simulink model "Impedance"  (R2021a)
settings: Solver=VariableStepAuto  StartTime=0.0  StopTime=2  RelTol=1e-3
values from neighbouring files (symbols this model uses):
  kd = 2*z*w    [params.m]
  kp = w^2    [params.m]
  Md = eye(6)*100    [params.m]
  x = [ 0.5357 ... (first row only)    [params.m]
settings Model: Creator=Sebastiano  LastModifiedBy=antoninoparisi
settings SolverCC: AlgebraicLoopSolver=TrustRegion
settings DebuggingCC: SFMachineParentedDataDiag=warning

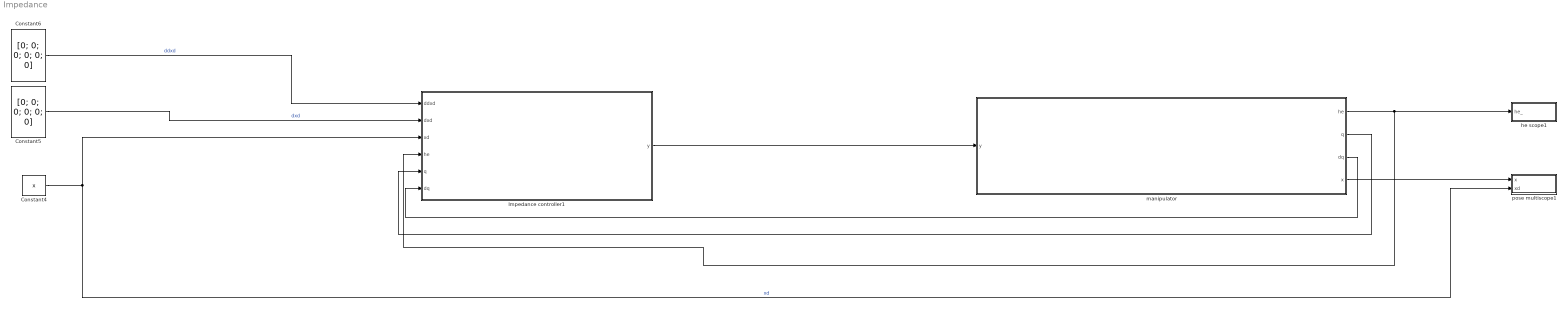
== system Impedance ==
  Constant4 : Constant  Value=x  VectorParams1D=off
  Constant5 : Constant  Value=[0; 0; 0; 0; 0; 0]  VectorParams1D=off
  Constant6 : Constant  Value=[0; 0; 0; 0; 0; 0]  VectorParams1D=off
  Impedance controller1 : Subsystem
  he scope1 : Subsystem
  manipulator : Subsystem
  pose multiscope1 : Subsystem
  wires:
  Constant5/1 -> Impedance controller1/2(dxd)  "dxd"
  manipulator/1(he) -> he scope1/1(he_), Impedance controller1/4(he)
  manipulator/3(dq) -> Impedance controller1/6(dq)
  Constant6/1 -> Impedance controller1/1(ddxd)  "ddxd"
  manipulator/2(q) -> Impedance controller1/5(q)
  manipulator/4(x) -> pose multiscope1/1(x)
  Constant4/1 -> Impedance controller1/3(xd), pose multiscope1/2(xd)  "xd"
  Impedance controller1/1(y) -> manipulator/1(y)

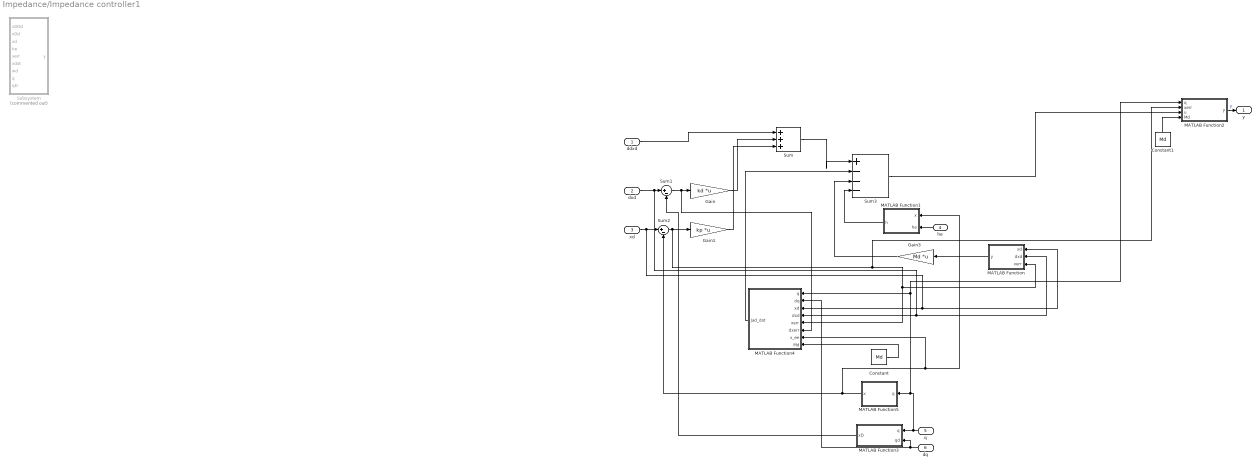
== system Impedance/Impedance controller1 ==
  ddxd : Inport
  dxd : Inport  Port=2
  xd : Inport  Port=3
  he : Inport  Port=4
  q : Inport  Port=5
  dq : Inport  Port=6
  Constant : Constant  Value=Md
  Constant1 : Constant  Value=Md
  Gain : Gain  Gain=kd  Multiplication=Matrix(K*u) (u vector)
  Gain1 : Gain  Gain=kp  Multiplication=Matrix(K*u) (u vector)
  Gain3 : Gain  Gain=Md  Multiplication=Matrix(K*u) (u vector)
  MATLAB Function : MATLAB Function  TreatAsAtomicUnit=on
  MATLAB Function1 : MATLAB Function  TreatAsAtomicUnit=on
  MATLAB Function2 : MATLAB Function  TreatAsAtomicUnit=on
  MATLAB Function3 : MATLAB Function  TreatAsAtomicUnit=on
  MATLAB Function4 : MATLAB Function  TreatAsAtomicUnit=on
  MATLAB Function5 : MATLAB Function  TreatAsAtomicUnit=on
  Subsystem : Subsystem  Commented=on
  Sum : Sum  Inputs=|+++
  Sum1 : Sum  Inputs=|+-
  Sum2 : Sum  Inputs=|+-
  Sum3 : Sum  Inputs=|+---
  y : Outport
  wires:
  xd/1 -> MATLAB Function/1(xd), MATLAB Function4/3(xd), Sum2/1
  Sum2/1 -> MATLAB Function/3(xerr), MATLAB Function4/5(xerr), MATLAB Function2/2(xerr), Gain1/1
  dxd/1 -> MATLAB Function/2(dxd), MATLAB Function4/4(dxd), Sum1/1
  Sum1/1 -> MATLAB Function4/6(dxerr), Gain/1
  ddxd/1 -> Sum/1
  Gain/1 -> Sum/2
  Gain1/1 -> Sum/3
  dq/1 -> MATLAB Function4/2(dq), MATLAB Function3/2(qd)
  q/1 -> MATLAB Function2/1(q), MATLAB Function4/1(q), MATLAB Function5/1(q), MATLAB Function3/1(q)
  MATLAB Function3/1(xD) -> Sum1/2
  MATLAB Function5/1(x) -> MATLAB Function4/7(x_ee), MATLAB Function1/1(x), Sum2/2
  Sum/1 -> Sum3/1
  Sum3/1 -> MATLAB Function2/3(u)
  MATLAB Function/1(y) -> Gain3/1
  MATLAB Function2/1(y) -> y/1  "y"
  MATLAB Function1/1(h) -> Sum3/4
  MATLAB Function4/1(Jad_dot) -> Sum3/2
  Gain3/1 -> Sum3/3
  he/1 -> MATLAB Function1/2(he)
  Constant/1 -> MATLAB Function4/8(Md)
  Constant1/1 -> MATLAB Function2/4(Md)

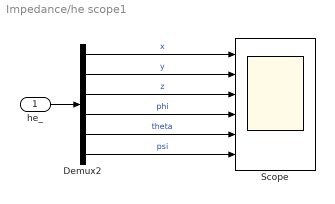
== system Impedance/he scope1 ==
  he_ : Inport
  Demux2 : Demux  Outputs=[1, 1, 1, 1, 1, 1]
  Scope : Scope  NumInputPorts=6
  wires:
  Demux2/4 -> Scope/4  "phi"
  Demux2/3 -> Scope/3  "z"
  Demux2/6 -> Scope/6  "psi"
  Demux2/5 -> Scope/5  "theta"
  Demux2/1 -> Scope/1  "x"
  he_/1 -> Demux2/1
  Demux2/2 -> Scope/2  "y"

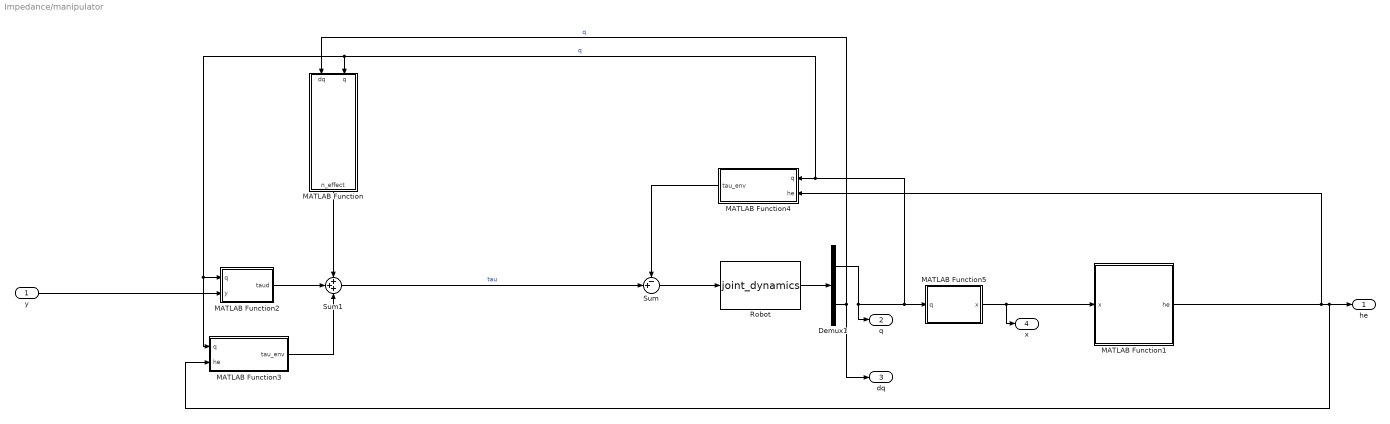
== system Impedance/manipulator ==
  y : Inport
  Demux1 : Demux  Outputs=[3, 3]
  MATLAB Function : MATLAB Function  TreatAsAtomicUnit=on
  MATLAB Function1 : MATLAB Function  TreatAsAtomicUnit=on
  MATLAB Function2 : MATLAB Function  TreatAsAtomicUnit=on
  MATLAB Function3 : MATLAB Function  TreatAsAtomicUnit=on
  MATLAB Function4 : MATLAB Function  TreatAsAtomicUnit=on
  MATLAB Function5 : MATLAB Function  TreatAsAtomicUnit=on
  Robot : S-Function  FunctionName=joint_dynamics  Parameters=robot  SFunctionDeploymentMode=off  EnableBusSupport=off
  Sum : Sum  Inputs=-+|
  Sum1 : Sum  Inputs=+++
  he : Outport
  q : Outport  Port=2
  dq : Outport  Port=3
  x : Outport  Port=4
  wires:
  Sum/1 -> Robot/1
  Robot/1 -> Demux1/1
  MATLAB Function4/1(tau_env) -> Sum/1
  MATLAB Function5/1(x) -> x/1, MATLAB Function1/1(x)
  MATLAB Function1/1(he) -> MATLAB Function4/2(he), MATLAB Function3/2(he), he/1
  Demux1/1 -> MATLAB Function5/1(q), MATLAB Function/2(q), MATLAB Function3/1(q), MATLAB Function2/1(q), MATLAB Function4/1(q), q/1  "q"
  y/1 -> MATLAB Function2/2(y)
  MATLAB Function/1(n_effect) -> Sum1/1
  Sum1/1 -> Sum/2  "tau"
  MATLAB Function3/1(tau_env) -> Sum1/3
  MATLAB Function2/1(taud) -> Sum1/2
  Demux1/2 -> dq/1, MATLAB Function/1(dq)  "q"

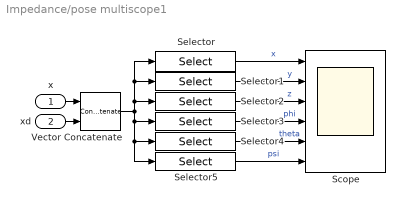
== system Impedance/pose multiscope1 ==
  x : Inport
  xd : Inport  Port=2
  Scope : Scope  NumInputPorts=6
  Selector : Selector  NumberOfDimensions=2  InputPortWidth=3  IndexOptions=Index vector (dialog),Select all  Indices=1,7  OutputSizes=6,6
  Selector1 : Selector  NumberOfDimensions=2  InputPortWidth=3  IndexOptions=Index vector (dialog),Select all  Indices=2,7  OutputSizes=6,6
  Selector2 : Selector  NumberOfDimensions=2  InputPortWidth=3  IndexOptions=Index vector (dialog),Select all  Indices=3,7  OutputSizes=6,6
  Selector3 : Selector  NumberOfDimensions=2  InputPortWidth=3  IndexOptions=Index vector (dialog),Select all  Indices=4,7  OutputSizes=6,6
  Selector4 : Selector  NumberOfDimensions=2  InputPortWidth=3  IndexOptions=Index vector (dialog),Select all  Indices=5,7  OutputSizes=6,6
  Selector5 : Selector  NumberOfDimensions=2  InputPortWidth=3  IndexOptions=Index vector (dialog),Select all  Indices=6,7  OutputSizes=6,6
  Vector Concatenate : Concatenate  Mode=Multidimensional array  ConcatenateDimension=2
  wires:
  x/1 -> Vector Concatenate/1
  xd/1 -> Vector Concatenate/2
  Selector1/1 -> Scope/2  "y"
  Selector5/1 -> Scope/6  "psi"
  Selector3/1 -> Scope/4  "phi"
  Selector/1 -> Scope/1  "x"
  Selector4/1 -> Scope/5  "theta"
  Vector Concatenate/1 -> Selector/1, Selector1/1, Selector2/1, Selector5/1, Selector4/1, Selector3/1
  Selector2/1 -> Scope/3  "z"

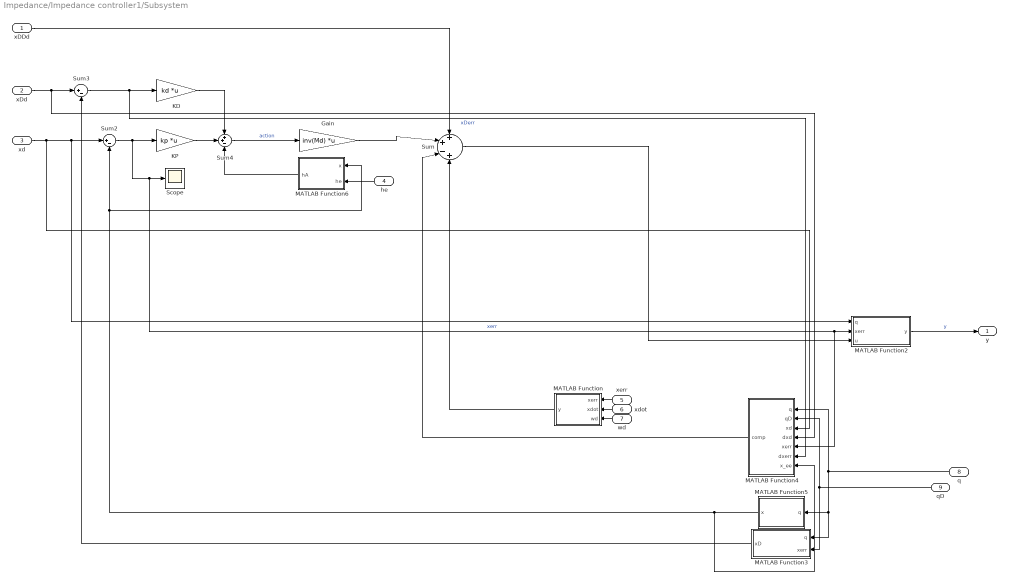
== system Impedance/Impedance controller1/Subsystem ==
  xDDd : Inport
  xDd : Inport  Port=2
  xd : Inport  Port=3
  he : Inport  Port=4
  xerr : Inport  Port=5
  xdot : Inport  Port=6
  wd : Inport  Port=7
  q : Inport  Port=8
  qD : Inport  Port=9
  Gain : Gain  Gain=inv(Md)  Multiplication=Matrix(K*u) (u vector)
  KD : Gain  Gain=kd  Multiplication=Matrix(K*u) (u vector)
  KP : Gain  Gain=kp  Multiplication=Matrix(K*u) (u vector)
  MATLAB Function : MATLAB Function  TreatAsAtomicUnit=on
  MATLAB Function2 : MATLAB Function  TreatAsAtomicUnit=on
  MATLAB Function3 : MATLAB Function  TreatAsAtomicUnit=on
  MATLAB Function4 : MATLAB Function  TreatAsAtomicUnit=on
  MATLAB Function5 : MATLAB Function  TreatAsAtomicUnit=on
  MATLAB Function6 : MATLAB Function  TreatAsAtomicUnit=on
  Scope : Scope
  Sum : Sum  Inputs=++-+
  Sum2 : Sum  Inputs=|+-
  Sum3 : Sum  Inputs=|+-
  Sum4 : Sum  Inputs=++-
  y : Outport
  wires:
  xdot/1 -> MATLAB Function/2(xdot)
  wd/1 -> MATLAB Function/3(wd)
  MATLAB Function/1(y) -> Sum/4
  he/1 -> MATLAB Function6/2(he)
  Sum4/1 -> Gain/1  "action"
  Gain/1 -> Sum/2
  xDDd/1 -> Sum/1
  MATLAB Function3/1(xD) -> Sum3/2
  KD/1 -> Sum4/1
  KP/1 -> Sum4/2
  xerr/1 -> MATLAB Function/1(xerr)
  MATLAB Function4/1(comp) -> Sum/3
  MATLAB Function2/1(y) -> y/1  "y"
  xDd/1 -> MATLAB Function4/4(dxd), Sum3/1
  qD/1 -> MATLAB Function4/2(qD), MATLAB Function3/2(xerr)
  MATLAB Function5/1(x) -> MATLAB Function4/7(x_ee), Sum2/2, MATLAB Function6/1(x)
  Sum/1 -> MATLAB Function2/3(u)
  Sum2/1 -> MATLAB Function2/2(xerr), MATLAB Function4/5(xerr), Scope/1, KP/1  "xerr"
  xd/1 -> MATLAB Function4/3(xd), MATLAB Function2/1(q), Sum2/1
  MATLAB Function6/1(hA) -> Sum4/3
  q/1 -> MATLAB Function4/1(q), MATLAB Function5/1(q), MATLAB Function3/1(q)
  Sum3/1 -> MATLAB Function4/6(dxerr), KD/1  "xDerr"

== matlab function Impedance/Impedance controller1/Subsystem/MATLAB Function5 ==
  data: q input; x output
function x = K(q)

t1 = q(1);
d1 = q(2);
t2 = q(3);


a1 = 0.15;
a2 = 0.4;
a3 = 0.3;
a4 = 0.16;


% wrt frame 0
K = [[cos(t1)*cos(t2), -cos(t1)*sin(t2), -sin(t1),      a2*cos(t1) + a4*cos(t1)*cos(t2)]
    [        sin(t2),          cos(t2),        0,                 a4*sin(t2) - d1 - a3]
    [cos(t2)*sin(t1), -sin(t1)*sin(t2),  cos(t1), a1 + a2*sin(t1) + a4*cos(t2)*sin(t1)]
    [              0,                0,        0,                                    1]];

pos = K(1:3, 4);
ori = rotm2eul(K(1:3,1:3), 'ZYZ')';

x = [pos; ori];

== matlab function Impedance/Impedance controller1/Subsystem/MATLAB Function6 ==
  data: x input; hA output; he input
function hA = TAT(x,he)

ori = x(4:6);
hA = T_analytical(ori)' * he;

== matlab function Impedance/manipulator/MATLAB Function ==
  data: dq input; q input; n_effect output
function n_effect = n(dq, q)

n_effect = C_Lagrangian(q, dq)*dq + G_Lagrangian(q);

== matlab function Impedance/manipulator/MATLAB Function1 ==
  data: x input; he output
function he = environment(x)

% environment params
K = diag([2 2 2 0.1 0.1 0.1])*10;    % stiffness
wall = 0.16; % constraint position w.r.t. frame 0 (it's y=-0.5 w.r.t. base frame)

if abs(x(3)) >= wall  % check is done in frame 0
    % touching the environment! constrained motion
    % set up the rest position frame
    % (basically, same orientation as ee but position is the contact point at the wall)
    xr = x;
    xr(3) = wall;
    % calculate the forces
    dx_re = x - xr;
    he = K * dx_re;
else
    % free motion
    he = zeros(6,1);
end

he = reshape(he,[6 1]);

== matlab function Impedance/manipulator/MATLAB Function2 ==
  data: q input; taud output; y input
function taud = B(q, y)

taud = B_Lagrangian(q)*y;

== matlab function Impedance/Impedance controller1/MATLAB Function4 ==
  data: q input; Jad_dot output; dq input; xd input; dxd input; xerr input; dxerr input; x_ee input; Md input
function Jad_dot = JA_dD(q, dq,xd,dxd,xerr,dxerr,x_ee,Md)



%%%%%%%%%%%%%%%%%

% J_ad computation

%%%%%%%%%%%%%%%%%
% 
% ori = xerr(4:6);
% 
% T = T_analytical(ori);
% 
% T_inv = pinv(T);
% 
% Ta = [eye(3),zeros(3);
%       zeros(3), T_inv];
% 
% Ta_inv = pinv(Ta);
% 
% Rd = eultorotm(ori,'ZYZ');
% 
% Rd_mtx = [ Rd',zeros(3);
%            zeros(3), Rd'];
% 
% J = jacobian(q);
% 
% 
% Jad = Ta_inv*Rd_mtx*J;


%%%%%%%%%%%%%%%%%

%end 

%%%%%%%%%%%%%%%%%


% part 1 Ta_dot_inv * Rd * J(q)
ori = xerr(4:6)';

T_dot = Tdot_analytical(ori);

T_dot_inv = pinv(T_dot);

Ta_dot = [zeros(3),zeros(3);
      zeros(3), T_dot_inv];

Ta_dot_inv = pinv(Ta_dot);





% part 2

% Ta_inv * (Rd_dot * J(q) + Rd *J_dot(q))
T = T_analytical_mtx(ori);

T_inv = pinv(T);

Ta = [eye(3),zeros(3);
      zeros(3), T_inv];

Ta_inv = pinv(Ta);

Rd = eul2rotm(ori,'ZYZ');

Rd_mtx = [ Rd',zeros(3);
           zeros(3), Rd'];

J = jacobian(q);
J_dot = jacobian_dot(q,dq);


w = dxerr(4:6);
S = S_rot(w);

Rd_dot = [ Rd'*S,zeros(3);
           zeros(3), Rd'*S];



Jad_dot = Md*(Ta_dot_inv * Rd_mtx * J  + Ta_inv * (Rd_dot * J + Rd_mtx * J_dot))*dq;

== matlab function Impedance/manipulator/MATLAB Function3 ==
  data: q input; he input; tau_env output
function tau_env = J(q, he)

tau_env = jacobian(q)' * he;

== matlab function Impedance/manipulator/MATLAB Function4 ==
  data: q input; he input; tau_env output
function tau_env = J(q, he)

tau_env = jacobian(q)' * he;

== matlab function Impedance/manipulator/MATLAB Function5 ==
  data: q input; x output
function x = K(q)

t1 = q(1);
d1 = q(2);
t2 = q(3);


a1 = 0.15;
a2 = 0.4;
a3 = 0.3;
a4 = 0.16;


% wrt frame 0
K = [[cos(t1)*cos(t2), -cos(t1)*sin(t2), -sin(t1),      a2*cos(t1) + a4*cos(t1)*cos(t2)]
    [        sin(t2),          cos(t2),        0,                 a4*sin(t2) - d1 - a3]
    [cos(t2)*sin(t1), -sin(t1)*sin(t2),  cos(t1), a1 + a2*sin(t1) + a4*cos(t2)*sin(t1)]
    [              0,                0,        0,                                    1]];

pos = K(1:3, 4);
ori = rotm2eul(K(1:3,1:3), 'ZYZ')';

x = [pos; ori];

== matlab function Impedance/Impedance controller1/Subsystem/MATLAB Function ==
  data: xerr input; y output; xdot input; wd input
function y = b(xerr,xdot,wd)

y = xerr;

== matlab function Impedance/Impedance controller1/MATLAB Function3 ==
  data: q input; xD output; qd input
function xD = JAd(q, qd)


xD = analyticalJacobian(q)*qd;

== matlab function Impedance/Impedance controller1/MATLAB Function5 ==
  data: q input; x output
function x = K(q)

t1 = q(1);
d1 = q(2);
t2 = q(3);


a1 = 0.15;
a2 = 0.4;
a3 = 0.3;
a4 = 0.16;


% wrt frame 0
K = [[cos(t1)*cos(t2), -cos(t1)*sin(t2), -sin(t1),      a2*cos(t1) + a4*cos(t1)*cos(t2)]
    [        sin(t2),          cos(t2),        0,                 a4*sin(t2) - d1 - a3]
    [cos(t2)*sin(t1), -sin(t1)*sin(t2),  cos(t1), a1 + a2*sin(t1) + a4*cos(t2)*sin(t1)]
    [              0,                0,        0,                                    1]];

pos = K(1:3, 4);
ori = rotm2eul(K(1:3,1:3), 'ZYZ')';

x = [pos; ori];

== matlab function Impedance/Impedance controller1/MATLAB Function2 ==
  data: q input; y output; xerr input; u input; Md input
function y = JA_d_inv(q,xerr, u,Md)


ori = xerr(4:6)';

T = T_analytical_mtx(ori);

T_inv = pinv(T);

Ta = [eye(3),zeros(3);
      zeros(3), T_inv];

Ta_inv = pinv(Ta);

Rd = eul2rotm(ori,'ZYZ');

Rd_mtx = [ Rd',zeros(3);
           zeros(3), Rd'];

J = jacobian(q);


Jad = Ta_inv*Rd_mtx*J;

y = pinv(Jad)*pinv(Md)*u;

== matlab function Impedance/Impedance controller1/MATLAB Function ==
  data: xd input; dxd input; xerr input; y output
function y = b(xd,dxd,xerr)

ori = xerr(4:6)';

Rd = eul2rotm(ori,'ZYZ');


w = dxd(4:6);
tmp1 = Rd'*dxd(4:6) + S_rot(w)*dxd(4:6);


T = T_analytical_mtx(ori);

T_inv = pinv(T);



tmp2 = pinv(T_inv)*w;


y = [ tmp1; tmp2];

== matlab function Impedance/Impedance controller1/MATLAB Function1 ==
  data: x input; h output; he input
function h = h_ed(x,he)

ori = x(4:6);
h = T_analytical(ori)' * he;

== matlab function Impedance/Impedance controller1/Subsystem/MATLAB Function2 ==
  data: q input; y output; xerr input; u input
function y = JA_d_inv(q,xerr,u)

y = pinv(analyticalJacobian(q)) * dq;

== matlab function Impedance/Impedance controller1/Subsystem/MATLAB Function3 ==
  data: q input; xD output; xerr input
function xD = JAd(q, xerr)

xD = analyticalJacobian(q)*qD;

== matlab function Impedance/Impedance controller1/Subsystem/MATLAB Function4 ==
  data: q input; comp output; qD input; xd input; dxd input; xerr input; dxerr input; x_ee input
function comp = JA_dD(q, qD,xd,dxd,xerr,dxerr,x_ee)

t1 = q(1);
d1 = q(2);
t2 = q(3);

Dt1 = qD(1);
Dt2 = qD(2);
Dd3 = qD(3);

a1 = 0.15;
a2 = 0.4;
a3 = 0.3;
a4 = 0.16;

JAD = [[- a4*cos(t1 + t2) - (pi*cos(t1))/100, 0,        -a4*cos(t1 + t2)]
[                                   0, 0,             -a4*sin(t2)]
[- a4*sin(t1 + t2) - (pi*sin(t1))/100, 0,        -a4*sin(t1 + t2)]
[                                   0, 0,                       0]
[                                   0, 0,                       0]
[                                   0, 0, -2^(1/2)*sin(t1 + pi/4)]];
comp = JAD*qD;
